simulink model "mainSimulink_localPi_B"  (R2021a)
settings: Solver=VariableStepAuto  StartTime=0.0  StopTime=inf  FixedStep=sensorSamplingTime  RelTol=1e-3
model workspace (MATLAB code in the model file):
  | %% Simulink settings
  | controllerFile = 'directFFcontroller';
  | set_param('mainSimulink_localPi_B/Subsystem Reference', 'ReferencedSubsystem', controllerFile);
  | %% Display settings
  | scopeTimeSpan = 30;
  | 
  | %% Robot settings (must match Python)
  | sensorFreq = 125;
  | actuatorFreq = 125;
  | TCPport = 12345;
  | dataSize = 4;
  | sensorSamplingTime = 1/sensorFreq;
  | actuatorTime = 1/actuatorFreq;
undefined symbols (not defined in the file): f
libraries: instrumentlib x2, simulink x1
settings Model: Creator=chukh  LastModifiedBy=brandon

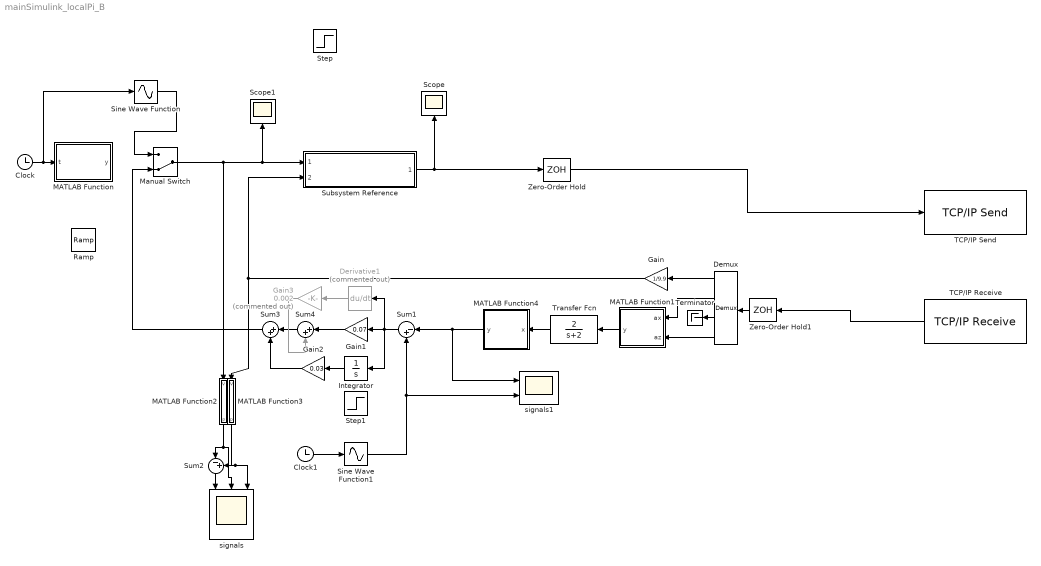
== system mainSimulink_localPi_B ==
  Clock : Clock
  Clock1 : Clock
  Demux : Demux
  Derivative1 : Derivative  Commented=on
  Gain : Gain  Gain=1/9.9
  Gain1 : Gain  Gain=0.07
  Gain2 : Gain  Gain=0.03
  Gain3 : Gain  Commented=on  Gain=0.002
  Integrator : Integrator
  MATLAB Function : MATLAB Function  TreatAsAtomicUnit=on
  MATLAB Function1 : MATLAB Function  TreatAsAtomicUnit=on
  MATLAB Function2 : MATLAB Function  TreatAsAtomicUnit=on
  MATLAB Function3 : MATLAB Function  TreatAsAtomicUnit=on
  MATLAB Function4 : MATLAB Function  TreatAsAtomicUnit=on
  Manual Switch : ManualSwitch  CurrentSetting=0
  Ramp : simulink/Sources/Ramp  slope=0.06  start=3  InitialOutput=0.6
  Scope : Scope
  Scope1 : Scope
  Sine Wave Function : Sin  TimeSource=Use external signal  Amplitude=.4  Bias=0.5  Frequency=2  SampleTime=0
  Sine Wave Function1 : Sin  TimeSource=Use external signal  Amplitude=6  Bias=5  Frequency=4  SampleTime=0
  Step : Step  Time=4  Before=0.6  After=0.85  SampleTime=0
  Step1 : Step  Time=4  After=10  SampleTime=0
  Subsystem Reference : Subsystem  ReferencedSubsystem=directFFcontroller
  Sum1 : Sum  Inputs=|-+
  Sum2 : Sum  Inputs=|-+
  Sum3 : Sum  Inputs=|++
  Sum4 : Sum  Inputs=|++
  TCP/IP Receive : instrumentlib/TCP//IP Receive  Host=server.softrobot  Port=TCPport  DataSize=dataSize  EnableBlockingMode=on  Timeout=0.5  SampleTime=sensorSamplingTime  DataType=double  ByteOrder=LittleEndian  ASCIIFormatting=%f,  Terminator=LF
  TCP/IP Send : instrumentlib/TCP//IP Send  Host=server.softrobot  Port=TCPport  EnableBlockingMode=on  Timeout=0.5  ByteOrder=LittleEndian  TransferDelay=on
  Terminator : Terminator
  Transfer Fcn : TransferFcn  Numerator=[2]  Denominator=[1 2]
  Zero-Order Hold : ZeroOrderHold  SampleTime=actuatorTime
  Zero-Order Hold1 : ZeroOrderHold  SampleTime=actuatorTime
  signals : Scope  NumInputPorts=3
  signals1 : Scope  NumInputPorts=2
  wires:
  Subsystem Reference/1 -> Zero-Order Hold/1, Scope/1
  TCP/IP Receive/1 -> Zero-Order Hold1/1
  Zero-Order Hold/1 -> TCP/IP Send/1
  MATLAB Function2/1(p) -> Sum2/1, signals/2
  Gain/1 -> MATLAB Function3/1(V), Subsystem Reference/2
  MATLAB Function3/1(p) -> Sum2/2, signals/3
  Sum2/1 -> signals/1
  Clock/1 -> Sine Wave Function/1, MATLAB Function/1(t)
  Manual Switch/1 -> Scope1/1, Subsystem Reference/1, MATLAB Function2/1(V)
  Sine Wave Function/1 -> Manual Switch/1
  Demux/1 -> Gain/1
  Zero-Order Hold1/1 -> Demux/1
  Demux/4 -> MATLAB Function1/2(az)
  Demux/2 -> MATLAB Function1/1(ax)
  MATLAB Function1/1(y) -> Transfer Fcn/1
  Demux/3 -> Terminator/1
  Transfer Fcn/1 -> MATLAB Function4/1(x)
  MATLAB Function4/1(y) -> Sum1/1, signals1/1
  Integrator/1 -> Gain2/1
  Gain2/1 -> Sum3/2
  Sum3/1 -> Manual Switch/2
  Clock1/1 -> Sine Wave Function1/1
  Sum1/1 -> Integrator/1, Derivative1/1, Gain1/1
  Sum4/1 -> Sum3/1
  Gain1/1 -> Sum4/1
  Derivative1/1 -> Gain3/1
  Gain3/1 -> Sum4/2
  Sine Wave Function1/1 -> Sum1/2, signals1/2

== matlab function mainSimulink_localPi_B/MATLAB Function2 ==
  data: V input; p output
function p = V2kPa(V)
p = (V-0.5)*200;

== matlab function mainSimulink_localPi_B/MATLAB Function3 ==
  data: V input; p output
function p = V2kPa(V)
p = (V-0.5)*200;

== matlab function mainSimulink_localPi_B/MATLAB Function1 ==
  data: ax input; y output; az input
function y = fcn(ax,az)

y = -atan2(-az,-ax);

== matlab function mainSimulink_localPi_B/MATLAB Function4 ==
  data: x input; y output
function y = rad2kappa(x)
y = x/0.0875;
end

== matlab function mainSimulink_localPi_B/MATLAB Function ==
  data: t input; y output
function y = fcn(t)

y = (0.6+0.3*sin(0.25*t^2));
